simulink model "Demo_CarRealTime2D_cs"  (R2014b)
settings: Solver=ode5  SolverMode=SingleTasking  StartTime=0.0  StopTime=inf  FixedStep=1/1000  RelTol=1e-3
PreLoadFcn:
  | mbxruntime.callbacks.PreLoadFcn(bdroot);
  | check_NUTS_defined;
  | assignin('base',['model_closed_' bdroot],false);
  | addpath('../includes_AEBS');
PostLoadFcn:
  | mbxruntime.callbacks.PostLoadFcn(bdroot);
InitFcn:
  | mbxruntime.callbacks.InitFcn(bdroot);
StartFcn:
  | mbxruntime.callbacks.StartFcn(bdroot);
StopFcn:
  | mbxruntime.callbacks.StopFcn(bdroot);;
  | 
model workspace: external: MAT-File .\Demo_CarRealTime2D_cs_hws.mat (data not in the file)
undefined symbols (not defined in the file or in its folder): Driver_Demands, mbxruntime, tabledata, vicrt_initcallback, vicrt_initmexcallback, vicrt_simulationmanager, warningInitialVelocity, x0
undefined symbols (not defined in the file): Demo_CarRealTime2D_cs_007c1c37f387f47f, Demo_CarRealTime2D_cs_085a64a83ba38cec, Demo_CarRealTime2D_cs_0a7f542d3fc7ab9f, Demo_CarRealTime2D_cs_0d7c72cfaa56dff7, Demo_CarRealTime2D_cs_0de07b35068e3828, Demo_CarRealTime2D_cs_17f4d381375cce95, Demo_CarRealTime2D_cs_1db40a09b08215a9, Demo_CarRealTime2D_cs_2bfa3850c176687b, Demo_CarRealTime2D_cs_35a34f1ba6ce4a22, Demo_CarRealTime2D_cs_378cc77e08d643fb, Demo_CarRealTime2D_cs_409b5c3befba0000, Demo_CarRealTime2D_cs_42628ca5bb62d2f3, Demo_CarRealTime2D_cs_56554a2db408a7f8, Demo_CarRealTime2D_cs_59527455249d7429, Demo_CarRealTime2D_cs_5983ee1b8112afac, Demo_CarRealTime2D_cs_5b5ebcf3ed7bf8e6, Demo_CarRealTime2D_cs_63cbe7fbe16cd5d9, Demo_CarRealTime2D_cs_6e17b9adbf989abf, Demo_CarRealTime2D_cs_6f662a34e5d9a196, Demo_CarRealTime2D_cs_75c4ee8892821e19, Demo_CarRealTime2D_cs_7c64486355814be2, Demo_CarRealTime2D_cs_849809550a2230ef, Demo_CarRealTime2D_cs_87f899bcbe16d8f5, Demo_CarRealTime2D_cs_8e7b50dac25b68a2, Demo_CarRealTime2D_cs_94938e5260f139b3, Demo_CarRealTime2D_cs_983acc940698d1d1, Demo_CarRealTime2D_cs_9d554c72797f76fd, Demo_CarRealTime2D_cs_9d747ee2f15c057f, Demo_CarRealTime2D_cs_ad62a2084d31e898, Demo_CarRealTime2D_cs_b56c8c5f000d30f0, Demo_CarRealTime2D_cs_b95f1b7356e926cc, Demo_CarRealTime2D_cs_BMW_X5_1_Path_pathUniqueID, Demo_CarRealTime2D_cs_BMW_Z3_2_Dynamics_Empty_STATE_BMW_Z3_2_x0, Demo_CarRealTime2D_cs_BMW_Z3_2_Dynamics_Empty_STATE_BMW_Z3_2_y0, Demo_CarRealTime2D_cs_BMW_Z3_2_Dynamics_Empty_STATE_BMW_Z3_2_z0, Demo_CarRealTime2D_cs_BMW_Z3_Path_pathUniqueID, Demo_CarRealTime2D_cs_BMW_Z3_SpeedProfile_speedProfileUniqueID, Demo_CarRealTime2D_cs_c8847ab2e5633224, Demo_CarRealTime2D_cs_c9a0d701286b93fb, Demo_CarRealTime2D_cs_ce758cae7dd1b283, Demo_CarRealTime2D_cs_CrossingPedestrian_Path_pathUniqueID, Demo_CarRealTime2D_cs_CuttingInVehicle_Path_pathUniqueID, Demo_CarRealTime2D_cs_d901ab1c1d2e40bc, Demo_CarRealTime2D_cs_dff70430e5a00a86, Demo_CarRealTime2D_cs_ef038a4f619ad32e, Demo_CarRealTime2D_cs_Female_OverweightAni_1_Path_pathUniqueID, Demo_CarRealTime2D_cs_Ford_Fiesta_1_Path_pathUniqueID, Demo_CarRealTime2D_cs_Ford_FocusWagon_Path_pathUniqueID, Demo_CarRealTime2D_cs_Sphere_1_Dynamics_Empty_STATE_Sphere_1_x0, Demo_CarRealTime2D_cs_Sphere_1_Dynamics_Empty_STATE_Sphere_1_y0, Demo_CarRealTime2D_cs_Sphere_1_Dynamics_Empty_STATE_Sphere_1_z0, WheelL0, WheelL1, WheelR0, WheelR1
libraries: PreScanSimulinkLibrary x15, simulink x15, simulink_extras x15, PreScanUsefulBlocks x2, dspsigops x1
(part 6 of 17)

== system Demo_CarRealTime2D_cs/Actros_2541_1/SELF_Demux ==
  SELF : Inport  OutDataTypeStr=Bus: PRESCAN_SELFSENSORDATA
  Bus Selector : BusSelector  OutputSignals=PositionX,PositionY,PositionZ,OrientationRoll,OrientationPitch,OrientationYaw,Velocity,Yaw_rate,Lat,Long,Alt
  Demux2 : Demux  Outputs=3
  Gain : Gain  Gain=180/pi
  Gain1 : Gain  Gain=180/pi
  Vector Concatenate1 : Concatenate  NumInputs=3
  compas converter : Subsystem
  x [m] : Outport
  y [m] : Outport  Port=2
  z [m] : Outport  Port=3
  rotx [deg] : Outport  Port=4
  roty [deg] : Outport  Port=5
  rotz [deg] : Outport  Port=6
  GPS lat [deg] : Outport  Port=7
  GPS long [deg] : Outport  Port=8
  GPS alt [m] : Outport  Port=9
  velocity [m/s] : Outport  Port=10
  heading [deg] : Outport  Port=11
  yaw rate [deg/s] : Outport  Port=12
  wires:
  Bus Selector/11 -> GPS alt [m]/1  "<Alt>"
  Bus Selector/10 -> GPS long [deg]/1  "<Long>"
  Bus Selector/9 -> GPS lat [deg]/1  "<Lat>"
  Bus Selector/8 -> Gain1/1  "<Yaw_rate>"
  Bus Selector/7 -> velocity [m/s]/1  "<Velocity>"
  Bus Selector/6 -> compas converter/1(rotz [rad]), Vector Concatenate1/3  "<OrientationYaw>"
  Bus Selector/5 -> Vector Concatenate1/2  "<OrientationPitch>"
  Bus Selector/4 -> Vector Concatenate1/1  "<OrientationRoll>"
  Vector Concatenate1/1 -> Gain/1
  Bus Selector/3 -> z [m]/1  "<PositionZ>"
  Bus Selector/2 -> y [m]/1  "<PositionY>"
  Bus Selector/1 -> x [m]/1  "<PositionX>"
  SELF/1 -> Bus Selector/1
  Gain/1 -> Demux2/1
  Demux2/1 -> rotx [deg]/1
  Demux2/2 -> roty [deg]/1
  Demux2/3 -> rotz [deg]/1
  compas converter/1(heading [deg]) -> heading [deg]/1
  Gain1/1 -> yaw rate [deg/s]/1

== system Demo_CarRealTime2D_cs/BMW_X5_1/JointGroup_WheelDisplacement_V2R ==
  Velocity [m/s] : Inport  SampleTime=TimeStep
  Discrete-Time Integrator : DiscreteIntegrator  SampleTime=TimeStep
  omega=V/Rwheel : Gain  Gain=1/TireRadius
  Rotation [rad] : Outport
  wires:
  Discrete-Time Integrator/1 -> Rotation [rad]/1  "roty"
  omega=V/Rwheel/1 -> Discrete-Time Integrator/1  "rotational speed [rad/s]"
  Velocity [m/s]/1 -> omega=V/Rwheel/1

== system Demo_CarRealTime2D_cs/BMW_X5_1/SELF_Demux ==
  SELF : Inport  OutDataTypeStr=Bus: PRESCAN_SELFSENSORDATA
  Bus Selector : BusSelector  OutputSignals=PositionX,PositionY,PositionZ,OrientationRoll,OrientationPitch,OrientationYaw,Velocity,Yaw_rate,Lat,Long,Alt
  Demux2 : Demux  Outputs=3
  Gain : Gain  Gain=180/pi
  Gain1 : Gain  Gain=180/pi
  Vector Concatenate1 : Concatenate  NumInputs=3
  compas converter : Subsystem
  x [m] : Outport
  y [m] : Outport  Port=2
  z [m] : Outport  Port=3
  rotx [deg] : Outport  Port=4
  roty [deg] : Outport  Port=5
  rotz [deg] : Outport  Port=6
  GPS lat [deg] : Outport  Port=7
  GPS long [deg] : Outport  Port=8
  GPS alt [m] : Outport  Port=9
  velocity [m/s] : Outport  Port=10
  heading [deg] : Outport  Port=11
  yaw rate [deg/s] : Outport  Port=12
  wires:
  Bus Selector/11 -> GPS alt [m]/1  "<Alt>"
  Bus Selector/10 -> GPS long [deg]/1  "<Long>"
  Bus Selector/9 -> GPS lat [deg]/1  "<Lat>"
  Bus Selector/8 -> Gain1/1  "<Yaw_rate>"
  Bus Selector/7 -> velocity [m/s]/1  "<Velocity>"
  Bus Selector/6 -> compas converter/1(rotz [rad]), Vector Concatenate1/3  "<OrientationYaw>"
  Bus Selector/5 -> Vector Concatenate1/2  "<OrientationPitch>"
  Bus Selector/4 -> Vector Concatenate1/1  "<OrientationRoll>"
  Vector Concatenate1/1 -> Gain/1
  Bus Selector/3 -> z [m]/1  "<PositionZ>"
  Bus Selector/2 -> y [m]/1  "<PositionY>"
  Bus Selector/1 -> x [m]/1  "<PositionX>"
  SELF/1 -> Bus Selector/1
  Gain/1 -> Demux2/1
  Demux2/1 -> rotx [deg]/1
  Demux2/2 -> roty [deg]/1
  Demux2/3 -> rotz [deg]/1
  compas converter/1(heading [deg]) -> heading [deg]/1
  Gain1/1 -> yaw rate [deg/s]/1

== system Demo_CarRealTime2D_cs/BMW_X5_1/WheelDisplacement_Mux ==
  Steering Angle Front [rad] : Inport  Tag=inport/JointGroup  SampleTime=10/1000  BusOutputAsStruct=on
  Steering Angle Rear [rad] : Inport  Tag=inport/JointGroup  Port=2  SampleTime=10/1000  BusOutputAsStruct=on
  Rotation [rad] : Inport  Tag=inport/JointGroup  Port=3  SampleTime=10/1000  BusOutputAsStruct=on
  zDisp FL [m] : Inport  Tag=inport/JointGroup  Port=4  SampleTime=10/1000  BusOutputAsStruct=on
  zDisp FR [m] : Inport  Tag=inport/JointGroup  Port=5  SampleTime=10/1000  BusOutputAsStruct=on
  zDisp RL [m] : Inport  Tag=inport/JointGroup  Port=6  SampleTime=10/1000  BusOutputAsStruct=on
  zDisp RR [m] : Inport  Tag=inport/JointGroup  Port=7  SampleTime=10/1000  BusOutputAsStruct=on
  Ground_{1..12} (12 alike) : Ground
  WheelL0_Mux : Subsystem  Tag=mux/Joint  mask(PreScan Mux Block){DisplayName=WheelL0}
      mask prompts: DisplayName "Display Name"
      mask help:
      | This block simulates a generic joint used for generic models. This joint can be enabled/disabled from the GUI.
      |
      | For more information, please click Help.
      settings: DeleteFcn=PreScanBlockDeleteFcn;
      mask Help: eval('openHelp(254)')
  WheelL1_Mux : Subsystem  Tag=mux/Joint  mask(PreScan Mux Block){DisplayName=WheelL1}
      mask prompts: DisplayName "Display Name"
      mask help:
      | This block simulates a generic joint used for generic models. This joint can be enabled/disabled from the GUI.
      |
      | For more information, please click Help.
      settings: DeleteFcn=PreScanBlockDeleteFcn;
      mask Help: eval('openHelp(254)')
  WheelR0_Mux : Subsystem  Tag=mux/Joint  mask(PreScan Mux Block){DisplayName=WheelR0}
      mask prompts: DisplayName "Display Name"
      mask help:
      | This block simulates a generic joint used for generic models. This joint can be enabled/disabled from the GUI.
      |
      | For more information, please click Help.
      settings: DeleteFcn=PreScanBlockDeleteFcn;
      mask Help: eval('openHelp(254)')
  WheelR1_Mux : Subsystem  Tag=mux/Joint  mask(PreScan Mux Block){DisplayName=WheelR1}
      mask prompts: DisplayName "Display Name"
      mask help:
      | This block simulates a generic joint used for generic models. This joint can be enabled/disabled from the GUI.
      |
      | For more information, please click Help.
      settings: DeleteFcn=PreScanBlockDeleteFcn;
      mask Help: eval('openHelp(254)')
  WheelL0_BMW_X5_1 : Outport  Tag=outport/JointActuator  OutDataTypeStr=Bus: PRESCAN_POSE_DATA  SampleTime=10/1000
  WheelR0_BMW_X5_1 : Outport  Tag=outport/JointActuator  Port=2  OutDataTypeStr=Bus: PRESCAN_POSE_DATA  SampleTime=10/1000
  WheelR1_BMW_X5_1 : Outport  Tag=outport/JointActuator  Port=3  OutDataTypeStr=Bus: PRESCAN_POSE_DATA  SampleTime=10/1000
  WheelL1_BMW_X5_1 : Outport  Tag=outport/JointActuator  Port=4  OutDataTypeStr=Bus: PRESCAN_POSE_DATA  SampleTime=10/1000
  wires:
  WheelL0_Mux/1(Joint) -> WheelL0_BMW_X5_1/1
  WheelR0_Mux/1(Joint) -> WheelR0_BMW_X5_1/1
  WheelR1_Mux/1(Joint) -> WheelR1_BMW_X5_1/1
  WheelL1_Mux/1(Joint) -> WheelL1_BMW_X5_1/1
  Steering Angle Front [rad]/1 -> WheelR0_Mux/6(Yaw [rad]), WheelL0_Mux/6(Yaw [rad])
  Steering Angle Rear [rad]/1 -> WheelR1_Mux/6(Yaw [rad]), WheelL1_Mux/6(Yaw [rad])
  Rotation [rad]/1 -> WheelR0_Mux/5(Pitch [rad]), WheelL0_Mux/5(Pitch [rad]), WheelR1_Mux/5(Pitch [rad]), WheelL1_Mux/5(Pitch [rad])
  zDisp FL [m]/1 -> WheelL0_Mux/3(Z [m])
  zDisp FR [m]/1 -> WheelR0_Mux/3(Z [m])
  zDisp RL [m]/1 -> WheelL1_Mux/3(Z [m])
  zDisp RR [m]/1 -> WheelR1_Mux/3(Z [m])
  Ground_1/1 -> WheelL0_Mux/1(X [m])
  Ground_2/1 -> WheelL0_Mux/2(Y [m])
  Ground_3/1 -> WheelL0_Mux/4(Roll [rad])
  Ground_4/1 -> WheelL1_Mux/1(X [m])
  Ground_5/1 -> WheelL1_Mux/2(Y [m])
  Ground_6/1 -> WheelL1_Mux/4(Roll [rad])
  Ground_7/1 -> WheelR0_Mux/1(X [m])
  Ground_8/1 -> WheelR0_Mux/2(Y [m])
  Ground_9/1 -> WheelR0_Mux/4(Roll [rad])
  Ground_10/1 -> WheelR1_Mux/1(X [m])
  Ground_11/1 -> WheelR1_Mux/2(Y [m])
  Ground_12/1 -> WheelR1_Mux/4(Roll [rad])

== system Demo_CarRealTime2D_cs/BMW_X5_1/d2r WheelDisplacement_Mux 1 ==
  Degrees in : Inport
  Gain1 : Gain  Gain=pi/180  SaturateOnIntegerOverflow=on  OutDataTypeStr=Inherit: Same as input  ParamDataTypeStr=Inherit: Same as input
  Radians out : Outport  InitialOutput=0
  wires:
  Gain1/1 -> Radians out/1
  Degrees in/1 -> Gain1/1

== system Demo_CarRealTime2D_cs/BMW_X5_1/d2r WheelDisplacement_Mux 2 ==
  Degrees in : Inport
  Gain1 : Gain  Gain=pi/180  SaturateOnIntegerOverflow=on  OutDataTypeStr=Inherit: Same as input  ParamDataTypeStr=Inherit: Same as input
  Radians out : Outport  InitialOutput=0
  wires:
  Gain1/1 -> Radians out/1
  Degrees in/1 -> Gain1/1

== system Demo_CarRealTime2D_cs/BMW_Z3/JointGroup_WheelDisplacement_V2R ==
  Velocity [m/s] : Inport  SampleTime=TimeStep
  Discrete-Time Integrator : DiscreteIntegrator  SampleTime=TimeStep
  omega=V/Rwheel : Gain  Gain=1/TireRadius
  Rotation [rad] : Outport
  wires:
  Discrete-Time Integrator/1 -> Rotation [rad]/1  "roty"
  omega=V/Rwheel/1 -> Discrete-Time Integrator/1  "rotational speed [rad/s]"
  Velocity [m/s]/1 -> omega=V/Rwheel/1

== system Demo_CarRealTime2D_cs/BMW_Z3/SELF_Demux ==
  SELF : Inport  OutDataTypeStr=Bus: PRESCAN_SELFSENSORDATA
  Bus Selector : BusSelector  OutputSignals=PositionX,PositionY,PositionZ,OrientationRoll,OrientationPitch,OrientationYaw,Velocity,Yaw_rate,Lat,Long,Alt
  Demux2 : Demux  Outputs=3
  Gain : Gain  Gain=180/pi
  Gain1 : Gain  Gain=180/pi
  Vector Concatenate1 : Concatenate  NumInputs=3
  compas converter : Subsystem
  x [m] : Outport
  y [m] : Outport  Port=2
  z [m] : Outport  Port=3
  rotx [deg] : Outport  Port=4
  roty [deg] : Outport  Port=5
  rotz [deg] : Outport  Port=6
  GPS lat [deg] : Outport  Port=7
  GPS long [deg] : Outport  Port=8
  GPS alt [m] : Outport  Port=9
  velocity [m/s] : Outport  Port=10
  heading [deg] : Outport  Port=11
  yaw rate [deg/s] : Outport  Port=12
  wires:
  Bus Selector/11 -> GPS alt [m]/1  "<Alt>"
  Bus Selector/10 -> GPS long [deg]/1  "<Long>"
  Bus Selector/9 -> GPS lat [deg]/1  "<Lat>"
  Bus Selector/8 -> Gain1/1  "<Yaw_rate>"
  Bus Selector/7 -> velocity [m/s]/1  "<Velocity>"
  Bus Selector/6 -> compas converter/1(rotz [rad]), Vector Concatenate1/3  "<OrientationYaw>"
  Bus Selector/5 -> Vector Concatenate1/2  "<OrientationPitch>"
  Bus Selector/4 -> Vector Concatenate1/1  "<OrientationRoll>"
  Vector Concatenate1/1 -> Gain/1
  Bus Selector/3 -> z [m]/1  "<PositionZ>"
  Bus Selector/2 -> y [m]/1  "<PositionY>"
  Bus Selector/1 -> x [m]/1  "<PositionX>"
  SELF/1 -> Bus Selector/1
  Gain/1 -> Demux2/1
  Demux2/1 -> rotx [deg]/1
  Demux2/2 -> roty [deg]/1
  Demux2/3 -> rotz [deg]/1
  compas converter/1(heading [deg]) -> heading [deg]/1
  Gain1/1 -> yaw rate [deg/s]/1

== system Demo_CarRealTime2D_cs/BMW_Z3/WheelDisplacement_Mux ==
  Steering Angle Front [rad] : Inport  Tag=inport/JointGroup  SampleTime=10/1000  BusOutputAsStruct=on
  Steering Angle Rear [rad] : Inport  Tag=inport/JointGroup  Port=2  SampleTime=10/1000  BusOutputAsStruct=on
  Rotation [rad] : Inport  Tag=inport/JointGroup  Port=3  SampleTime=10/1000  BusOutputAsStruct=on
  zDisp FL [m] : Inport  Tag=inport/JointGroup  Port=4  SampleTime=10/1000  BusOutputAsStruct=on
  zDisp FR [m] : Inport  Tag=inport/JointGroup  Port=5  SampleTime=10/1000  BusOutputAsStruct=on
  zDisp RL [m] : Inport  Tag=inport/JointGroup  Port=6  SampleTime=10/1000  BusOutputAsStruct=on
  zDisp RR [m] : Inport  Tag=inport/JointGroup  Port=7  SampleTime=10/1000  BusOutputAsStruct=on
  Ground_{1..12} (12 alike) : Ground
  WheelL0_Mux : Subsystem  Tag=mux/Joint  mask(PreScan Mux Block){DisplayName=WheelL0}
      mask prompts: DisplayName "Display Name"
      mask help:
      | This block simulates a generic joint used for generic models. This joint can be enabled/disabled from the GUI.
      |
      | For more information, please click Help.
      settings: DeleteFcn=PreScanBlockDeleteFcn;
      mask Help: eval('openHelp(254)')
  WheelL1_Mux : Subsystem  Tag=mux/Joint  mask(PreScan Mux Block){DisplayName=WheelL1}
      mask prompts: DisplayName "Display Name"
      mask help:
      | This block simulates a generic joint used for generic models. This joint can be enabled/disabled from the GUI.
      |
      | For more information, please click Help.
      settings: DeleteFcn=PreScanBlockDeleteFcn;
      mask Help: eval('openHelp(254)')
  WheelR0_Mux : Subsystem  Tag=mux/Joint  mask(PreScan Mux Block){DisplayName=WheelR0}
      mask prompts: DisplayName "Display Name"
      mask help:
      | This block simulates a generic joint used for generic models. This joint can be enabled/disabled from the GUI.
      |
      | For more information, please click Help.
      settings: DeleteFcn=PreScanBlockDeleteFcn;
      mask Help: eval('openHelp(254)')
  WheelR1_Mux : Subsystem  Tag=mux/Joint  mask(PreScan Mux Block){DisplayName=WheelR1}
      mask prompts: DisplayName "Display Name"
      mask help:
      | This block simulates a generic joint used for generic models. This joint can be enabled/disabled from the GUI.
      |
      | For more information, please click Help.
      settings: DeleteFcn=PreScanBlockDeleteFcn;
      mask Help: eval('openHelp(254)')
  WheelL0_BMW_Z3 : Outport  Tag=outport/JointActuator  OutDataTypeStr=Bus: PRESCAN_POSE_DATA  SampleTime=10/1000
  WheelL1_BMW_Z3 : Outport  Tag=outport/JointActuator  Port=2  OutDataTypeStr=Bus: PRESCAN_POSE_DATA  SampleTime=10/1000
  WheelR0_BMW_Z3 : Outport  Tag=outport/JointActuator  Port=3  OutDataTypeStr=Bus: PRESCAN_POSE_DATA  SampleTime=10/1000
  WheelR1_BMW_Z3 : Outport  Tag=outport/JointActuator  Port=4  OutDataTypeStr=Bus: PRESCAN_POSE_DATA  SampleTime=10/1000
  wires:
  WheelL0_Mux/1(Joint) -> WheelL0_BMW_Z3/1
  WheelL1_Mux/1(Joint) -> WheelL1_BMW_Z3/1
  WheelR0_Mux/1(Joint) -> WheelR0_BMW_Z3/1
  WheelR1_Mux/1(Joint) -> WheelR1_BMW_Z3/1
  Steering Angle Front [rad]/1 -> WheelR0_Mux/6(Yaw [rad]), WheelL0_Mux/6(Yaw [rad])
  Steering Angle Rear [rad]/1 -> WheelR1_Mux/6(Yaw [rad]), WheelL1_Mux/6(Yaw [rad])
  Rotation [rad]/1 -> WheelR0_Mux/5(Pitch [rad]), WheelL0_Mux/5(Pitch [rad]), WheelR1_Mux/5(Pitch [rad]), WheelL1_Mux/5(Pitch [rad])
  zDisp FL [m]/1 -> WheelL0_Mux/3(Z [m])
  zDisp FR [m]/1 -> WheelR0_Mux/3(Z [m])
  zDisp RL [m]/1 -> WheelL1_Mux/3(Z [m])
  zDisp RR [m]/1 -> WheelR1_Mux/3(Z [m])
  Ground_1/1 -> WheelL0_Mux/1(X [m])
  Ground_2/1 -> WheelL0_Mux/2(Y [m])
  Ground_3/1 -> WheelL0_Mux/4(Roll [rad])
  Ground_4/1 -> WheelL1_Mux/1(X [m])
  Ground_5/1 -> WheelL1_Mux/2(Y [m])
  Ground_6/1 -> WheelL1_Mux/4(Roll [rad])
  Ground_7/1 -> WheelR0_Mux/1(X [m])
  Ground_8/1 -> WheelR0_Mux/2(Y [m])
  Ground_9/1 -> WheelR0_Mux/4(Roll [rad])
  Ground_10/1 -> WheelR1_Mux/1(X [m])
  Ground_11/1 -> WheelR1_Mux/2(Y [m])
  Ground_12/1 -> WheelR1_Mux/4(Roll [rad])

== system Demo_CarRealTime2D_cs/BMW_Z3/d2r WheelDisplacement_Mux 1 ==
  Degrees in : Inport
  Gain1 : Gain  Gain=pi/180  SaturateOnIntegerOverflow=on  OutDataTypeStr=Inherit: Same as input  ParamDataTypeStr=Inherit: Same as input
  Radians out : Outport  InitialOutput=0
  wires:
  Gain1/1 -> Radians out/1
  Degrees in/1 -> Gain1/1

== system Demo_CarRealTime2D_cs/BMW_Z3/d2r WheelDisplacement_Mux 2 ==
  Degrees in : Inport
  Gain1 : Gain  Gain=pi/180  SaturateOnIntegerOverflow=on  OutDataTypeStr=Inherit: Same as input  ParamDataTypeStr=Inherit: Same as input
  Radians out : Outport  InitialOutput=0
  wires:
  Gain1/1 -> Radians out/1
  Degrees in/1 -> Gain1/1

== system Demo_CarRealTime2D_cs/BMW_Z3_2/Dynamics_Empty ==
  note: For state mode 'Dynamic' positions
      | are not taken into account, as they
      | are computed by integrating velocity.
      | Click annotation for Help.
  Ground_{1..9} (9 alike) : Ground
  MuxState : Subsystem  Tag=mux/State  mask(Empty Dynamics State Block){positioningmode=on, TimeStep=1/1000}
      mask prompts: positioningmode "Positioning Mode"; TimeStep "Auto Assigned: Time Step [s]"
      mask help:
      | Build the state of an actor based on user input.
      | The user can either use positioning mode or dynamics mode.
      | - When using positioning mode the position and orientation of the actor are set directly based on the input. Expected input is relative to the initial position and orientation of the actor. It's also possible to specify the velocity of the actor, though this input isn't used, only passed on.
      | - When using dynamics mode the position input is ignored. Expected input is velocity and orientation. The velocity is relative the current orientation of the actor, while orientation is relative to its initial orientation. The position of the actor is calculated based on the velocity and orientation given.
      settings: DeleteFcn=PreScanBlockDeleteFcn;
  STATE_BMW_Z3_2 : Subsystem  Tag=mux/StatePort  Priority=0  LoadFcn=load PrescanStateActuatorData  mask(PreScan Sink Block: State){x0=Demo_CarRealTime2D_cs_BMW_Z3_2_Dynamics_Empty_STATE_BMW_Z3_2_x0, y0=Demo_CarRealTime2D_cs_BMW_Z3_2_Dynamics_Empty_STATE_BMW_Z3_2_y0, z0=Demo_CarRealTime2D_cs_BMW_Z3_2_Dynamics_Empty_STATE_BMW_Z3_2_z0, Roll0=Demo_CarRealTime2D_cs_d901ab1c1d2e40bc, Pitch0=Demo_CarRealTime2D_cs_ef038a4f619ad32e, Yaw0=Demo_CarRealTime2D_cs_6e17b9adbf989abf, TimeStep=1/1000}
      mask prompts: x0 "Ini x-position VEHICLE wrt GLOBAL axis system [m]"; y0 "Ini y-position VEHICLE wrt GLOBAL axis system [m]"; z0 "Ini z-position VEHICLE wrt GLOBAL axis system [m]"; Roll0 "Ini roll-angle BODY wrt VEHICLE axis system [deg]"; Pitch0 "Ini pitch-angle BODY wrt VEHICLE axis system [deg]"; Yaw0 "Ini yaw-angle VEHICLE wrt GLOBAL axis system [deg]"; TimeStep "Auto-Assigned: Upload Period [s]"
      mask help:
      | The Actor State contains a vector signal of size (9x1), containing the following signals:
      |
      | -  Position                  (x,y,z)                                     [m]
      | -  Velocity                  (vx,vy,vz)                               [m/s]
      | -  Angles                    (Roll, Pitch, Yaw)                   [rad]
      |
      | The Actor state is defined in the global axis system.
      | The state is superponed on the Initial position defined in the GUI.
      |
      | For more information, please click Help.
      settings: DeleteFcn=PreScanBlockDeleteFcn;
      mask Help: eval('openHelp(222)')
      mask Display: image(imread('State.png'))
  State : Outport  Tag=outport/StateOutport  SampleTime=1/1000
  wires:
  MuxState/1(state) -> STATE_BMW_Z3_2/1(State)
  STATE_BMW_Z3_2/1(StateBus) -> State/1
  Ground_1/1 -> MuxState/1(x [m])
  Ground_2/1 -> MuxState/2(y [m])
  Ground_3/1 -> MuxState/3(z [m])
  Ground_4/1 -> MuxState/4(dx [m/s])
  Ground_5/1 -> MuxState/5(dy [m/s])
  Ground_6/1 -> MuxState/6(dz [m/s])
  Ground_7/1 -> MuxState/7(R [rad])
  Ground_8/1 -> MuxState/8(P [rad])
  Ground_9/1 -> MuxState/9(Y [rad])

== system Demo_CarRealTime2D_cs/BMW_Z3_2/SELF_Demux ==
  SELF : Inport  OutDataTypeStr=Bus: PRESCAN_SELFSENSORDATA
  Bus Selector : BusSelector  OutputSignals=PositionX,PositionY,PositionZ,OrientationRoll,OrientationPitch,OrientationYaw,Velocity,Yaw_rate,Lat,Long,Alt
  Demux2 : Demux  Outputs=3
  Gain : Gain  Gain=180/pi
  Gain1 : Gain  Gain=180/pi
  Vector Concatenate1 : Concatenate  NumInputs=3
  compas converter : Subsystem
  x [m] : Outport
  y [m] : Outport  Port=2
  z [m] : Outport  Port=3
  rotx [deg] : Outport  Port=4
  roty [deg] : Outport  Port=5
  rotz [deg] : Outport  Port=6
  GPS lat [deg] : Outport  Port=7
  GPS long [deg] : Outport  Port=8
  GPS alt [m] : Outport  Port=9
  velocity [m/s] : Outport  Port=10
  heading [deg] : Outport  Port=11
  yaw rate [deg/s] : Outport  Port=12
  wires:
  Bus Selector/11 -> GPS alt [m]/1  "<Alt>"
  Bus Selector/10 -> GPS long [deg]/1  "<Long>"
  Bus Selector/9 -> GPS lat [deg]/1  "<Lat>"
  Bus Selector/8 -> Gain1/1  "<Yaw_rate>"
  Bus Selector/7 -> velocity [m/s]/1  "<Velocity>"
  Bus Selector/6 -> compas converter/1(rotz [rad]), Vector Concatenate1/3  "<OrientationYaw>"
  Bus Selector/5 -> Vector Concatenate1/2  "<OrientationPitch>"
  Bus Selector/4 -> Vector Concatenate1/1  "<OrientationRoll>"
  Vector Concatenate1/1 -> Gain/1
  Bus Selector/3 -> z [m]/1  "<PositionZ>"
  Bus Selector/2 -> y [m]/1  "<PositionY>"
  Bus Selector/1 -> x [m]/1  "<PositionX>"
  SELF/1 -> Bus Selector/1
  Gain/1 -> Demux2/1
  Demux2/1 -> rotx [deg]/1
  Demux2/2 -> roty [deg]/1
  Demux2/3 -> rotz [deg]/1
  compas converter/1(heading [deg]) -> heading [deg]/1
  Gain1/1 -> yaw rate [deg/s]/1

== system Demo_CarRealTime2D_cs/CrossingPedestrian/Animation ==
  In1 : Inport
  Bus Creator : BusCreator  Inputs=2  OutDataTypeStr=Bus: PRESCAN_ANIMACTUATORDATA  NonVirtualBus=on
  Bus Selector : BusSelector  OutputSignals=VelocityX,VelocityY,VelocityZ
  Data Type Conversion : DataTypeConversion  OutDataTypeStr=int32
  Mux : Mux  Inputs=3
  Product : Product  RndMeth=Zero
  RunningScale : Constant  Value=RunningScale
  Switch : Switch  Threshold=2
  WalkingScale : Constant  Value=WalkingScale
  animation mode : Subsystem
  elapsed track : Subsystem
  Out1 : Outport
  wires:
  Switch/1 -> Product/1
  WalkingScale/1 -> Switch/3
  RunningScale/1 -> Switch/1
  elapsed track/1(s) -> Product/2  "Time"
  Product/1 -> Bus Creator/2  "Time"
  Mux/1 -> elapsed track/1(vel), animation mode/1(vel)
  Bus Selector/1 -> Mux/1  "<VelocityX>"
  Bus Selector/2 -> Mux/2  "<VelocityY>"
  Bus Selector/3 -> Mux/3  "<VelocityZ>"
  animation mode/1(mode) -> Switch/2, Data Type Conversion/1
  In1/1 -> Bus Selector/1
  Bus Creator/1 -> Out1/1
  Data Type Conversion/1 -> Bus Creator/1  "Index"

== system Demo_CarRealTime2D_cs/CrossingPedestrian/SELF_Demux ==
  SELF : Inport  OutDataTypeStr=Bus: PRESCAN_SELFSENSORDATA
  Bus Selector : BusSelector  OutputSignals=PositionX,PositionY,PositionZ,OrientationRoll,OrientationPitch,OrientationYaw,Velocity,Yaw_rate,Lat,Long,Alt
  Demux2 : Demux  Outputs=3
  Gain : Gain  Gain=180/pi
  Gain1 : Gain  Gain=180/pi
  Vector Concatenate1 : Concatenate  NumInputs=3
  compas converter : Subsystem
  x [m] : Outport
  y [m] : Outport  Port=2
  z [m] : Outport  Port=3
  rotx [deg] : Outport  Port=4
  roty [deg] : Outport  Port=5
  rotz [deg] : Outport  Port=6
  GPS lat [deg] : Outport  Port=7
  GPS long [deg] : Outport  Port=8
  GPS alt [m] : Outport  Port=9
  velocity [m/s] : Outport  Port=10
  heading [deg] : Outport  Port=11
  yaw rate [deg/s] : Outport  Port=12
  wires:
  Bus Selector/11 -> GPS alt [m]/1  "<Alt>"
  Bus Selector/10 -> GPS long [deg]/1  "<Long>"
  Bus Selector/9 -> GPS lat [deg]/1  "<Lat>"
  Bus Selector/8 -> Gain1/1  "<Yaw_rate>"
  Bus Selector/7 -> velocity [m/s]/1  "<Velocity>"
  Bus Selector/6 -> compas converter/1(rotz [rad]), Vector Concatenate1/3  "<OrientationYaw>"
  Bus Selector/5 -> Vector Concatenate1/2  "<OrientationPitch>"
  Bus Selector/4 -> Vector Concatenate1/1  "<OrientationRoll>"
  Vector Concatenate1/1 -> Gain/1
  Bus Selector/3 -> z [m]/1  "<PositionZ>"
  Bus Selector/2 -> y [m]/1  "<PositionY>"
  Bus Selector/1 -> x [m]/1  "<PositionX>"
  SELF/1 -> Bus Selector/1
  Gain/1 -> Demux2/1
  Demux2/1 -> rotx [deg]/1
  Demux2/2 -> roty [deg]/1
  Demux2/3 -> rotz [deg]/1
  compas converter/1(heading [deg]) -> heading [deg]/1
  Gain1/1 -> yaw rate [deg/s]/1

== system Demo_CarRealTime2D_cs/CrossingPedestrian/VISUColorRegion_Lower_Body_Mux ==
  RGB [-,-,-] : Inport
  Bus Creator : BusCreator  OutDataTypeStr=Bus: PRESCAN_COLOR_DATA  NonVirtualBus=on
  Constant : Constant  Value=255  OutDataTypeStr=uint8
  Data Type Conversion : DataTypeConversion  OutDataTypeStr=uint8
  Data Type Conversion1 : DataTypeConversion  OutDataTypeStr=uint8
  Data Type Conversion2 : DataTypeConversion  OutDataTypeStr=uint8
  Demux : Demux  Outputs=3
  ColorRegion : Outport  OutDataTypeStr=Bus: PRESCAN_COLOR_DATA  PortDimensions=1
  wires:
  Constant/1 -> Bus Creator/4  "A"
  Data Type Conversion2/1 -> Bus Creator/3  "B"
  Data Type Conversion1/1 -> Bus Creator/2  "G"
  Data Type Conversion/1 -> Bus Creator/1  "R"
  Demux/3 -> Data Type Conversion2/1  "B"
  Demux/2 -> Data Type Conversion1/1  "G"
  Demux/1 -> Data Type Conversion/1  "R"
  RGB [-,-,-]/1 -> Demux/1
  Bus Creator/1 -> ColorRegion/1

== system Demo_CarRealTime2D_cs/CrossingPedestrian/VISUColorRegion_Shoes_Mux ==
  RGB [-,-,-] : Inport
  Bus Creator : BusCreator  OutDataTypeStr=Bus: PRESCAN_COLOR_DATA  NonVirtualBus=on
  Constant : Constant  Value=255  OutDataTypeStr=uint8
  Data Type Conversion : DataTypeConversion  OutDataTypeStr=uint8
  Data Type Conversion1 : DataTypeConversion  OutDataTypeStr=uint8
  Data Type Conversion2 : DataTypeConversion  OutDataTypeStr=uint8
  Demux : Demux  Outputs=3
  ColorRegion : Outport  OutDataTypeStr=Bus: PRESCAN_COLOR_DATA  PortDimensions=1
  wires:
  Constant/1 -> Bus Creator/4  "A"
  Data Type Conversion2/1 -> Bus Creator/3  "B"
  Data Type Conversion1/1 -> Bus Creator/2  "G"
  Data Type Conversion/1 -> Bus Creator/1  "R"
  Demux/3 -> Data Type Conversion2/1  "B"
  Demux/2 -> Data Type Conversion1/1  "G"
  Demux/1 -> Data Type Conversion/1  "R"
  RGB [-,-,-]/1 -> Demux/1
  Bus Creator/1 -> ColorRegion/1

== system Demo_CarRealTime2D_cs/CrossingPedestrian/VISUColorRegion_Upper_Body_Mux ==
  RGB [-,-,-] : Inport
  Bus Creator : BusCreator  OutDataTypeStr=Bus: PRESCAN_COLOR_DATA  NonVirtualBus=on
  Constant : Constant  Value=255  OutDataTypeStr=uint8
  Data Type Conversion : DataTypeConversion  OutDataTypeStr=uint8
  Data Type Conversion1 : DataTypeConversion  OutDataTypeStr=uint8
  Data Type Conversion2 : DataTypeConversion  OutDataTypeStr=uint8
  Demux : Demux  Outputs=3
  ColorRegion : Outport  OutDataTypeStr=Bus: PRESCAN_COLOR_DATA  PortDimensions=1
  wires:
  Constant/1 -> Bus Creator/4  "A"
  Data Type Conversion2/1 -> Bus Creator/3  "B"
  Data Type Conversion1/1 -> Bus Creator/2  "G"
  Data Type Conversion/1 -> Bus Creator/1  "R"
  Demux/3 -> Data Type Conversion2/1  "B"
  Demux/2 -> Data Type Conversion1/1  "G"
  Demux/1 -> Data Type Conversion/1  "R"
  RGB [-,-,-]/1 -> Demux/1
  Bus Creator/1 -> ColorRegion/1

== system Demo_CarRealTime2D_cs/CuttingInVehicle/JointGroup_WheelDisplacement_V2R ==
  Velocity [m/s] : Inport  SampleTime=TimeStep
  Discrete-Time Integrator : DiscreteIntegrator  SampleTime=TimeStep
  omega=V/Rwheel : Gain  Gain=1/TireRadius
  Rotation [rad] : Outport
  wires:
  Discrete-Time Integrator/1 -> Rotation [rad]/1  "roty"
  omega=V/Rwheel/1 -> Discrete-Time Integrator/1  "rotational speed [rad/s]"
  Velocity [m/s]/1 -> omega=V/Rwheel/1

== system Demo_CarRealTime2D_cs/CuttingInVehicle/MO_Path_0 ==
  In1 : Inport
  Constant : Constant
  Stop Simulation : Stop
  Terminator : Terminator
  wires:
  In1/1 -> Terminator/1
  Constant/1 -> Stop Simulation/1

== system Demo_CarRealTime2D_cs/CuttingInVehicle/SELF_Demux ==
  SELF : Inport  OutDataTypeStr=Bus: PRESCAN_SELFSENSORDATA
  Bus Selector : BusSelector  OutputSignals=PositionX,PositionY,PositionZ,OrientationRoll,OrientationPitch,OrientationYaw,Velocity,Yaw_rate,Lat,Long,Alt
  Demux2 : Demux  Outputs=3
  Gain : Gain  Gain=180/pi
  Gain1 : Gain  Gain=180/pi
  Vector Concatenate1 : Concatenate  NumInputs=3
  compas converter : Subsystem
  x [m] : Outport
  y [m] : Outport  Port=2
  z [m] : Outport  Port=3
  rotx [deg] : Outport  Port=4
  roty [deg] : Outport  Port=5
  rotz [deg] : Outport  Port=6
  GPS lat [deg] : Outport  Port=7
  GPS long [deg] : Outport  Port=8
  GPS alt [m] : Outport  Port=9
  velocity [m/s] : Outport  Port=10
  heading [deg] : Outport  Port=11
  yaw rate [deg/s] : Outport  Port=12
  wires:
  Bus Selector/11 -> GPS alt [m]/1  "<Alt>"
  Bus Selector/10 -> GPS long [deg]/1  "<Long>"
  Bus Selector/9 -> GPS lat [deg]/1  "<Lat>"
  Bus Selector/8 -> Gain1/1  "<Yaw_rate>"
  Bus Selector/7 -> velocity [m/s]/1  "<Velocity>"
  Bus Selector/6 -> compas converter/1(rotz [rad]), Vector Concatenate1/3  "<OrientationYaw>"
  Bus Selector/5 -> Vector Concatenate1/2  "<OrientationPitch>"
  Bus Selector/4 -> Vector Concatenate1/1  "<OrientationRoll>"
  Vector Concatenate1/1 -> Gain/1
  Bus Selector/3 -> z [m]/1  "<PositionZ>"
  Bus Selector/2 -> y [m]/1  "<PositionY>"
  Bus Selector/1 -> x [m]/1  "<PositionX>"
  SELF/1 -> Bus Selector/1
  Gain/1 -> Demux2/1
  Demux2/1 -> rotx [deg]/1
  Demux2/2 -> roty [deg]/1
  Demux2/3 -> rotz [deg]/1
  compas converter/1(heading [deg]) -> heading [deg]/1
  Gain1/1 -> yaw rate [deg/s]/1

== system Demo_CarRealTime2D_cs/CuttingInVehicle/Trajectories1 ==
  gain : Inport
  offset : Inport  Port=2
  Traj2State1 : Subsystem  Tag=Traj2State  mask(PreScan Demux Block:){}
      settings: DeleteFcn=PreScanBlockDeleteFcn;
  Trajectory_1_Offset : Constant  Tag=TrajectoryOffset  Value="[0  0  0  0  0  0]"
  Trajectory_Host_AllSystems : Subsystem  Tag=Trajectory  mask(PreScan Source Block: Trajectory){FileName='Trajectory_CuttingInVehicle.mat', TimeStep=1/40}
      mask prompts: TimeStep "Time Step [s]"
      mask help:
      | The Trajectory block contains the trajectories defined in the PreScan Experiment Editor. The output of the trajectory block is the (vehicle) State.
      |
      | For more information, please click Help.
      mask init:
      | [direc,name]=fileparts(get_param(bdroot, 'FileName'));
      | load([direc,'/Trajectories/',FileName])
      | trajectory=trajectory';
      | 
      | traj.time=trajectory(:,1);%[];
      | traj.signals.values=trajectory(:,2:19);
      | traj.dimensions=18;
      | traj.label='';
      | 
      | SampleTime=traj.time(2)-traj.time(1);
      settings: DeleteFcn=PreScanBlockDeleteFcn;
      mask Help: eval('openHelp(312)')
      mask Display: fprintf(FileName)
  State : Outport  Tag=TrajOutport
  wires:
  gain/1 -> Trajectory_Host_AllSystems/1(gain)
  offset/1 -> Trajectory_Host_AllSystems/2(offset)
  Trajectory_Host_AllSystems/1(trajectory) -> Traj2State1/1(Traj Org)  "L2"
  Trajectory_1_Offset/1 -> Traj2State1/2(Offset)  "L3"
  Traj2State1/1(state) -> State/1  "L4"

== system Demo_CarRealTime2D_cs/CuttingInVehicle/WheelDisplacement_Mux ==
  Steering Angle Front [rad] : Inport  Tag=inport/JointGroup  SampleTime=10/1000  BusOutputAsStruct=on
  Steering Angle Rear [rad] : Inport  Tag=inport/JointGroup  Port=2  SampleTime=10/1000  BusOutputAsStruct=on
  Rotation [rad] : Inport  Tag=inport/JointGroup  Port=3  SampleTime=10/1000  BusOutputAsStruct=on
  zDisp FL [m] : Inport  Tag=inport/JointGroup  Port=4  SampleTime=10/1000  BusOutputAsStruct=on
  zDisp FR [m] : Inport  Tag=inport/JointGroup  Port=5  SampleTime=10/1000  BusOutputAsStruct=on
  zDisp RL [m] : Inport  Tag=inport/JointGroup  Port=6  SampleTime=10/1000  BusOutputAsStruct=on
  zDisp RR [m] : Inport  Tag=inport/JointGroup  Port=7  SampleTime=10/1000  BusOutputAsStruct=on
  Ground_{1..12} (12 alike) : Ground
  WheelL0_Mux : Subsystem  Tag=mux/Joint  mask(PreScan Mux Block){DisplayName=WheelL0}
      mask prompts: DisplayName "Display Name"
      mask help:
      | This block simulates a generic joint used for generic models. This joint can be enabled/disabled from the GUI.
      |
      | For more information, please click Help.
      settings: DeleteFcn=PreScanBlockDeleteFcn;
      mask Help: eval('openHelp(254)')
  WheelL1_Mux : Subsystem  Tag=mux/Joint  mask(PreScan Mux Block){DisplayName=WheelL1}
      mask prompts: DisplayName "Display Name"
      mask help:
      | This block simulates a generic joint used for generic models. This joint can be enabled/disabled from the GUI.
      |
      | For more information, please click Help.
      settings: DeleteFcn=PreScanBlockDeleteFcn;
      mask Help: eval('openHelp(254)')
  WheelR0_Mux : Subsystem  Tag=mux/Joint  mask(PreScan Mux Block){DisplayName=WheelR0}
      mask prompts: DisplayName "Display Name"
      mask help:
      | This block simulates a generic joint used for generic models. This joint can be enabled/disabled from the GUI.
      |
      | For more information, please click Help.
      settings: DeleteFcn=PreScanBlockDeleteFcn;
      mask Help: eval('openHelp(254)')
  WheelR1_Mux : Subsystem  Tag=mux/Joint  mask(PreScan Mux Block){DisplayName=WheelR1}
      mask prompts: DisplayName "Display Name"
      mask help:
      | This block simulates a generic joint used for generic models. This joint can be enabled/disabled from the GUI.
      |
      | For more information, please click Help.
      settings: DeleteFcn=PreScanBlockDeleteFcn;
      mask Help: eval('openHelp(254)')
  WheelL0_CuttingInVehicle : Outport  Tag=outport/JointActuator  OutDataTypeStr=Bus: PRESCAN_POSE_DATA  SampleTime=10/1000
  WheelL1_CuttingInVehicle : Outport  Tag=outport/JointActuator  Port=2  OutDataTypeStr=Bus: PRESCAN_POSE_DATA  SampleTime=10/1000
  WheelR0_CuttingInVehicle : Outport  Tag=outport/JointActuator  Port=3  OutDataTypeStr=Bus: PRESCAN_POSE_DATA  SampleTime=10/1000
  WheelR1_CuttingInVehicle : Outport  Tag=outport/JointActuator  Port=4  OutDataTypeStr=Bus: PRESCAN_POSE_DATA  SampleTime=10/1000
  wires:
  WheelL0_Mux/1(Joint) -> WheelL0_CuttingInVehicle/1
  WheelL1_Mux/1(Joint) -> WheelL1_CuttingInVehicle/1
  WheelR0_Mux/1(Joint) -> WheelR0_CuttingInVehicle/1
  WheelR1_Mux/1(Joint) -> WheelR1_CuttingInVehicle/1
  Steering Angle Front [rad]/1 -> WheelR0_Mux/6(Yaw [rad]), WheelL0_Mux/6(Yaw [rad])
  Steering Angle Rear [rad]/1 -> WheelR1_Mux/6(Yaw [rad]), WheelL1_Mux/6(Yaw [rad])
  Rotation [rad]/1 -> WheelR0_Mux/5(Pitch [rad]), WheelL0_Mux/5(Pitch [rad]), WheelR1_Mux/5(Pitch [rad]), WheelL1_Mux/5(Pitch [rad])
  zDisp FL [m]/1 -> WheelL0_Mux/3(Z [m])
  zDisp FR [m]/1 -> WheelR0_Mux/3(Z [m])
  zDisp RL [m]/1 -> WheelL1_Mux/3(Z [m])
  zDisp RR [m]/1 -> WheelR1_Mux/3(Z [m])
  Ground_1/1 -> WheelL0_Mux/1(X [m])
  Ground_2/1 -> WheelL0_Mux/2(Y [m])
  Ground_3/1 -> WheelL0_Mux/4(Roll [rad])
  Ground_4/1 -> WheelL1_Mux/1(X [m])
  Ground_5/1 -> WheelL1_Mux/2(Y [m])
  Ground_6/1 -> WheelL1_Mux/4(Roll [rad])
  Ground_7/1 -> WheelR0_Mux/1(X [m])
  Ground_8/1 -> WheelR0_Mux/2(Y [m])
  Ground_9/1 -> WheelR0_Mux/4(Roll [rad])
  Ground_10/1 -> WheelR1_Mux/1(X [m])
  Ground_11/1 -> WheelR1_Mux/2(Y [m])
  Ground_12/1 -> WheelR1_Mux/4(Roll [rad])

== system Demo_CarRealTime2D_cs/CuttingInVehicle/d2r WheelDisplacement_Mux 1 ==
  Degrees in : Inport
  Gain1 : Gain  Gain=pi/180  SaturateOnIntegerOverflow=on  OutDataTypeStr=Inherit: Same as input  ParamDataTypeStr=Inherit: Same as input
  Radians out : Outport  InitialOutput=0
  wires:
  Gain1/1 -> Radians out/1
  Degrees in/1 -> Gain1/1

== system Demo_CarRealTime2D_cs/CuttingInVehicle/d2r WheelDisplacement_Mux 2 ==
  Degrees in : Inport
  Gain1 : Gain  Gain=pi/180  SaturateOnIntegerOverflow=on  OutDataTypeStr=Inherit: Same as input  ParamDataTypeStr=Inherit: Same as input
  Radians out : Outport  InitialOutput=0
  wires:
  Gain1/1 -> Radians out/1
  Degrees in/1 -> Gain1/1

== system Demo_CarRealTime2D_cs/Female_OverweightAni_1/Animation ==
  In1 : Inport
  Bus Creator : BusCreator  Inputs=2  OutDataTypeStr=Bus: PRESCAN_ANIMACTUATORDATA  NonVirtualBus=on
  Bus Selector : BusSelector  OutputSignals=VelocityX,VelocityY,VelocityZ
  Mux : Mux  Inputs=3
  animation mode : Subsystem
  elapsed track : Subsystem
  Out1 : Outport
  wires:
  animation mode/1(mode) -> Bus Creator/1  "Index"
  Bus Creator/1 -> Out1/1
  In1/1 -> Bus Selector/1
  elapsed track/1(s) -> Bus Creator/2  "Time"
  Bus Selector/3 -> Mux/3  "<VelocityZ>"
  Bus Selector/2 -> Mux/2  "<VelocityY>"
  Bus Selector/1 -> Mux/1  "<VelocityX>"
  Mux/1 -> animation mode/1(vel), elapsed track/1(vel)

== system Demo_CarRealTime2D_cs/Female_OverweightAni_1/SELF_Demux ==
  SELF : Inport  OutDataTypeStr=Bus: PRESCAN_SELFSENSORDATA
  Bus Selector : BusSelector  OutputSignals=PositionX,PositionY,PositionZ,OrientationRoll,OrientationPitch,OrientationYaw,Velocity,Yaw_rate,Lat,Long,Alt
  Demux2 : Demux  Outputs=3
  Gain : Gain  Gain=180/pi
  Gain1 : Gain  Gain=180/pi
  Vector Concatenate1 : Concatenate  NumInputs=3
  compas converter : Subsystem
  x [m] : Outport
  y [m] : Outport  Port=2
  z [m] : Outport  Port=3
  rotx [deg] : Outport  Port=4
  roty [deg] : Outport  Port=5
  rotz [deg] : Outport  Port=6
  GPS lat [deg] : Outport  Port=7
  GPS long [deg] : Outport  Port=8
  GPS alt [m] : Outport  Port=9
  velocity [m/s] : Outport  Port=10
  heading [deg] : Outport  Port=11
  yaw rate [deg/s] : Outport  Port=12
  wires:
  Bus Selector/11 -> GPS alt [m]/1  "<Alt>"
  Bus Selector/10 -> GPS long [deg]/1  "<Long>"
  Bus Selector/9 -> GPS lat [deg]/1  "<Lat>"
  Bus Selector/8 -> Gain1/1  "<Yaw_rate>"
  Bus Selector/7 -> velocity [m/s]/1  "<Velocity>"
  Bus Selector/6 -> compas converter/1(rotz [rad]), Vector Concatenate1/3  "<OrientationYaw>"
  Bus Selector/5 -> Vector Concatenate1/2  "<OrientationPitch>"
  Bus Selector/4 -> Vector Concatenate1/1  "<OrientationRoll>"
  Vector Concatenate1/1 -> Gain/1
  Bus Selector/3 -> z [m]/1  "<PositionZ>"
  Bus Selector/2 -> y [m]/1  "<PositionY>"
  Bus Selector/1 -> x [m]/1  "<PositionX>"
  SELF/1 -> Bus Selector/1
  Gain/1 -> Demux2/1
  Demux2/1 -> rotx [deg]/1
  Demux2/2 -> roty [deg]/1
  Demux2/3 -> rotz [deg]/1
  compas converter/1(heading [deg]) -> heading [deg]/1
  Gain1/1 -> yaw rate [deg/s]/1

== system Demo_CarRealTime2D_cs/Female_OverweightAni_1/VISUColorRegion_Lower_Body_Mux ==
  RGB [-,-,-] : Inport
  Bus Creator : BusCreator  OutDataTypeStr=Bus: PRESCAN_COLOR_DATA  NonVirtualBus=on
  Constant : Constant  Value=255  OutDataTypeStr=uint8
  Data Type Conversion : DataTypeConversion  OutDataTypeStr=uint8
  Data Type Conversion1 : DataTypeConversion  OutDataTypeStr=uint8
  Data Type Conversion2 : DataTypeConversion  OutDataTypeStr=uint8
  Demux : Demux  Outputs=3
  ColorRegion : Outport  OutDataTypeStr=Bus: PRESCAN_COLOR_DATA  PortDimensions=1
  wires:
  Constant/1 -> Bus Creator/4  "A"
  Data Type Conversion2/1 -> Bus Creator/3  "B"
  Data Type Conversion1/1 -> Bus Creator/2  "G"
  Data Type Conversion/1 -> Bus Creator/1  "R"
  Demux/3 -> Data Type Conversion2/1  "B"
  Demux/2 -> Data Type Conversion1/1  "G"
  Demux/1 -> Data Type Conversion/1  "R"
  RGB [-,-,-]/1 -> Demux/1
  Bus Creator/1 -> ColorRegion/1

== system Demo_CarRealTime2D_cs/Female_OverweightAni_1/VISUColorRegion_Shoes_Mux ==
  RGB [-,-,-] : Inport
  Bus Creator : BusCreator  OutDataTypeStr=Bus: PRESCAN_COLOR_DATA  NonVirtualBus=on
  Constant : Constant  Value=255  OutDataTypeStr=uint8
  Data Type Conversion : DataTypeConversion  OutDataTypeStr=uint8
  Data Type Conversion1 : DataTypeConversion  OutDataTypeStr=uint8
  Data Type Conversion2 : DataTypeConversion  OutDataTypeStr=uint8
  Demux : Demux  Outputs=3
  ColorRegion : Outport  OutDataTypeStr=Bus: PRESCAN_COLOR_DATA  PortDimensions=1
  wires:
  Constant/1 -> Bus Creator/4  "A"
  Data Type Conversion2/1 -> Bus Creator/3  "B"
  Data Type Conversion1/1 -> Bus Creator/2  "G"
  Data Type Conversion/1 -> Bus Creator/1  "R"
  Demux/3 -> Data Type Conversion2/1  "B"
  Demux/2 -> Data Type Conversion1/1  "G"
  Demux/1 -> Data Type Conversion/1  "R"
  RGB [-,-,-]/1 -> Demux/1
  Bus Creator/1 -> ColorRegion/1

== system Demo_CarRealTime2D_cs/Female_OverweightAni_1/VISUColorRegion_Upper_Body_Mux ==
  RGB [-,-,-] : Inport
  Bus Creator : BusCreator  OutDataTypeStr=Bus: PRESCAN_COLOR_DATA  NonVirtualBus=on
  Constant : Constant  Value=255  OutDataTypeStr=uint8
  Data Type Conversion : DataTypeConversion  OutDataTypeStr=uint8
  Data Type Conversion1 : DataTypeConversion  OutDataTypeStr=uint8
  Data Type Conversion2 : DataTypeConversion  OutDataTypeStr=uint8
  Demux : Demux  Outputs=3
  ColorRegion : Outport  OutDataTypeStr=Bus: PRESCAN_COLOR_DATA  PortDimensions=1
  wires:
  Constant/1 -> Bus Creator/4  "A"
  Data Type Conversion2/1 -> Bus Creator/3  "B"
  Data Type Conversion1/1 -> Bus Creator/2  "G"
  Data Type Conversion/1 -> Bus Creator/1  "R"
  Demux/3 -> Data Type Conversion2/1  "B"
  Demux/2 -> Data Type Conversion1/1  "G"
  Demux/1 -> Data Type Conversion/1  "R"
  RGB [-,-,-]/1 -> Demux/1
  Bus Creator/1 -> ColorRegion/1

== system Demo_CarRealTime2D_cs/Ford_Fiesta_1/JointGroup_WheelDisplacement_V2R ==
  Velocity [m/s] : Inport  SampleTime=TimeStep
  Discrete-Time Integrator : DiscreteIntegrator  SampleTime=TimeStep
  omega=V/Rwheel : Gain  Gain=1/TireRadius
  Rotation [rad] : Outport
  wires:
  Discrete-Time Integrator/1 -> Rotation [rad]/1  "roty"
  omega=V/Rwheel/1 -> Discrete-Time Integrator/1  "rotational speed [rad/s]"
  Velocity [m/s]/1 -> omega=V/Rwheel/1

== system Demo_CarRealTime2D_cs/Ford_Fiesta_1/SELF_Demux ==
  SELF : Inport  OutDataTypeStr=Bus: PRESCAN_SELFSENSORDATA
  Bus Selector : BusSelector  OutputSignals=PositionX,PositionY,PositionZ,OrientationRoll,OrientationPitch,OrientationYaw,Velocity,Yaw_rate,Lat,Long,Alt
  Demux2 : Demux  Outputs=3
  Gain : Gain  Gain=180/pi
  Gain1 : Gain  Gain=180/pi
  Vector Concatenate1 : Concatenate  NumInputs=3
  compas converter : Subsystem
  x [m] : Outport
  y [m] : Outport  Port=2
  z [m] : Outport  Port=3
  rotx [deg] : Outport  Port=4
  roty [deg] : Outport  Port=5
  rotz [deg] : Outport  Port=6
  GPS lat [deg] : Outport  Port=7
  GPS long [deg] : Outport  Port=8
  GPS alt [m] : Outport  Port=9
  velocity [m/s] : Outport  Port=10
  heading [deg] : Outport  Port=11
  yaw rate [deg/s] : Outport  Port=12
  wires:
  Bus Selector/11 -> GPS alt [m]/1  "<Alt>"
  Bus Selector/10 -> GPS long [deg]/1  "<Long>"
  Bus Selector/9 -> GPS lat [deg]/1  "<Lat>"
  Bus Selector/8 -> Gain1/1  "<Yaw_rate>"
  Bus Selector/7 -> velocity [m/s]/1  "<Velocity>"
  Bus Selector/6 -> compas converter/1(rotz [rad]), Vector Concatenate1/3  "<OrientationYaw>"
  Bus Selector/5 -> Vector Concatenate1/2  "<OrientationPitch>"
  Bus Selector/4 -> Vector Concatenate1/1  "<OrientationRoll>"
  Vector Concatenate1/1 -> Gain/1
  Bus Selector/3 -> z [m]/1  "<PositionZ>"
  Bus Selector/2 -> y [m]/1  "<PositionY>"
  Bus Selector/1 -> x [m]/1  "<PositionX>"
  SELF/1 -> Bus Selector/1
  Gain/1 -> Demux2/1
  Demux2/1 -> rotx [deg]/1
  Demux2/2 -> roty [deg]/1
  Demux2/3 -> rotz [deg]/1
  compas converter/1(heading [deg]) -> heading [deg]/1
  Gain1/1 -> yaw rate [deg/s]/1

== system Demo_CarRealTime2D_cs/Ford_Fiesta_1/WheelDisplacement_Mux ==
  Steering Angle Front [rad] : Inport  Tag=inport/JointGroup  SampleTime=10/1000  BusOutputAsStruct=on
  Steering Angle Rear [rad] : Inport  Tag=inport/JointGroup  Port=2  SampleTime=10/1000  BusOutputAsStruct=on
  Rotation [rad] : Inport  Tag=inport/JointGroup  Port=3  SampleTime=10/1000  BusOutputAsStruct=on
  zDisp FL [m] : Inport  Tag=inport/JointGroup  Port=4  SampleTime=10/1000  BusOutputAsStruct=on
  zDisp FR [m] : Inport  Tag=inport/JointGroup  Port=5  SampleTime=10/1000  BusOutputAsStruct=on
  zDisp RL [m] : Inport  Tag=inport/JointGroup  Port=6  SampleTime=10/1000  BusOutputAsStruct=on
  zDisp RR [m] : Inport  Tag=inport/JointGroup  Port=7  SampleTime=10/1000  BusOutputAsStruct=on
  Ground_{1..12} (12 alike) : Ground
  WheelL0_Mux : Subsystem  Tag=mux/Joint  mask(PreScan Mux Block){DisplayName=WheelL0}
      mask prompts: DisplayName "Display Name"
      mask help:
      | This block simulates a generic joint used for generic models. This joint can be enabled/disabled from the GUI.
      |
      | For more information, please click Help.
      settings: DeleteFcn=PreScanBlockDeleteFcn;
      mask Help: eval('openHelp(254)')
  WheelL1_Mux : Subsystem  Tag=mux/Joint  mask(PreScan Mux Block){DisplayName=WheelL1}
      mask prompts: DisplayName "Display Name"
      mask help:
      | This block simulates a generic joint used for generic models. This joint can be enabled/disabled from the GUI.
      |
      | For more information, please click Help.
      settings: DeleteFcn=PreScanBlockDeleteFcn;
      mask Help: eval('openHelp(254)')
  WheelR0_Mux : Subsystem  Tag=mux/Joint  mask(PreScan Mux Block){DisplayName=WheelR0}
      mask prompts: DisplayName "Display Name"
      mask help:
      | This block simulates a generic joint used for generic models. This joint can be enabled/disabled from the GUI.
      |
      | For more information, please click Help.
      settings: DeleteFcn=PreScanBlockDeleteFcn;
      mask Help: eval('openHelp(254)')
  WheelR1_Mux : Subsystem  Tag=mux/Joint  mask(PreScan Mux Block){DisplayName=WheelR1}
      mask prompts: DisplayName "Display Name"
      mask help:
      | This block simulates a generic joint used for generic models. This joint can be enabled/disabled from the GUI.
      |
      | For more information, please click Help.
      settings: DeleteFcn=PreScanBlockDeleteFcn;
      mask Help: eval('openHelp(254)')
  WheelL0_Ford_Fiesta_1 : Outport  Tag=outport/JointActuator  OutDataTypeStr=Bus: PRESCAN_POSE_DATA  SampleTime=10/1000
  WheelL1_Ford_Fiesta_1 : Outport  Tag=outport/JointActuator  Port=2  OutDataTypeStr=Bus: PRESCAN_POSE_DATA  SampleTime=10/1000
  WheelR0_Ford_Fiesta_1 : Outport  Tag=outport/JointActuator  Port=3  OutDataTypeStr=Bus: PRESCAN_POSE_DATA  SampleTime=10/1000
  WheelR1_Ford_Fiesta_1 : Outport  Tag=outport/JointActuator  Port=4  OutDataTypeStr=Bus: PRESCAN_POSE_DATA  SampleTime=10/1000
  wires:
  WheelL0_Mux/1(Joint) -> WheelL0_Ford_Fiesta_1/1
  WheelL1_Mux/1(Joint) -> WheelL1_Ford_Fiesta_1/1
  WheelR0_Mux/1(Joint) -> WheelR0_Ford_Fiesta_1/1
  WheelR1_Mux/1(Joint) -> WheelR1_Ford_Fiesta_1/1
  Steering Angle Front [rad]/1 -> WheelR0_Mux/6(Yaw [rad]), WheelL0_Mux/6(Yaw [rad])
  Steering Angle Rear [rad]/1 -> WheelR1_Mux/6(Yaw [rad]), WheelL1_Mux/6(Yaw [rad])
  Rotation [rad]/1 -> WheelR0_Mux/5(Pitch [rad]), WheelL0_Mux/5(Pitch [rad]), WheelR1_Mux/5(Pitch [rad]), WheelL1_Mux/5(Pitch [rad])
  zDisp FL [m]/1 -> WheelL0_Mux/3(Z [m])
  zDisp FR [m]/1 -> WheelR0_Mux/3(Z [m])
  zDisp RL [m]/1 -> WheelL1_Mux/3(Z [m])
  zDisp RR [m]/1 -> WheelR1_Mux/3(Z [m])
  Ground_1/1 -> WheelL0_Mux/1(X [m])
  Ground_2/1 -> WheelL0_Mux/2(Y [m])
  Ground_3/1 -> WheelL0_Mux/4(Roll [rad])
  Ground_4/1 -> WheelL1_Mux/1(X [m])
  Ground_5/1 -> WheelL1_Mux/2(Y [m])
  Ground_6/1 -> WheelL1_Mux/4(Roll [rad])
  Ground_7/1 -> WheelR0_Mux/1(X [m])
  Ground_8/1 -> WheelR0_Mux/2(Y [m])
  Ground_9/1 -> WheelR0_Mux/4(Roll [rad])
  Ground_10/1 -> WheelR1_Mux/1(X [m])
  Ground_11/1 -> WheelR1_Mux/2(Y [m])
  Ground_12/1 -> WheelR1_Mux/4(Roll [rad])

== system Demo_CarRealTime2D_cs/Ford_Fiesta_1/d2r WheelDisplacement_Mux 1 ==
  Degrees in : Inport
  Gain1 : Gain  Gain=pi/180  SaturateOnIntegerOverflow=on  OutDataTypeStr=Inherit: Same as input  ParamDataTypeStr=Inherit: Same as input
  Radians out : Outport  InitialOutput=0
  wires:
  Gain1/1 -> Radians out/1
  Degrees in/1 -> Gain1/1

== system Demo_CarRealTime2D_cs/Ford_Fiesta_1/d2r WheelDisplacement_Mux 2 ==
  Degrees in : Inport
  Gain1 : Gain  Gain=pi/180  SaturateOnIntegerOverflow=on  OutDataTypeStr=Inherit: Same as input  ParamDataTypeStr=Inherit: Same as input
  Radians out : Outport  InitialOutput=0
  wires:
  Gain1/1 -> Radians out/1
  Degrees in/1 -> Gain1/1

== system Demo_CarRealTime2D_cs/Ford_FocusWagon/JointGroup_WheelDisplacement_V2R ==
  Velocity [m/s] : Inport  SampleTime=TimeStep
  Discrete-Time Integrator : DiscreteIntegrator  SampleTime=TimeStep
  omega=V/Rwheel : Gain  Gain=1/TireRadius
  Rotation [rad] : Outport
  wires:
  Discrete-Time Integrator/1 -> Rotation [rad]/1  "roty"
  omega=V/Rwheel/1 -> Discrete-Time Integrator/1  "rotational speed [rad/s]"
  Velocity [m/s]/1 -> omega=V/Rwheel/1
